simulink subsystem "GravityTorque"  (R2021a)
settings: Solver=VariableStepAuto  StartTime=0.0  StopTime=10.0  RelTol=1e-3
undefined symbols (not defined in the file): Isc, Ix, Iy, Iz, mu
libraries: aerolibutil x2, vrlib x1
settings Model: Creator=Laura  LastModifiedBy=Laura

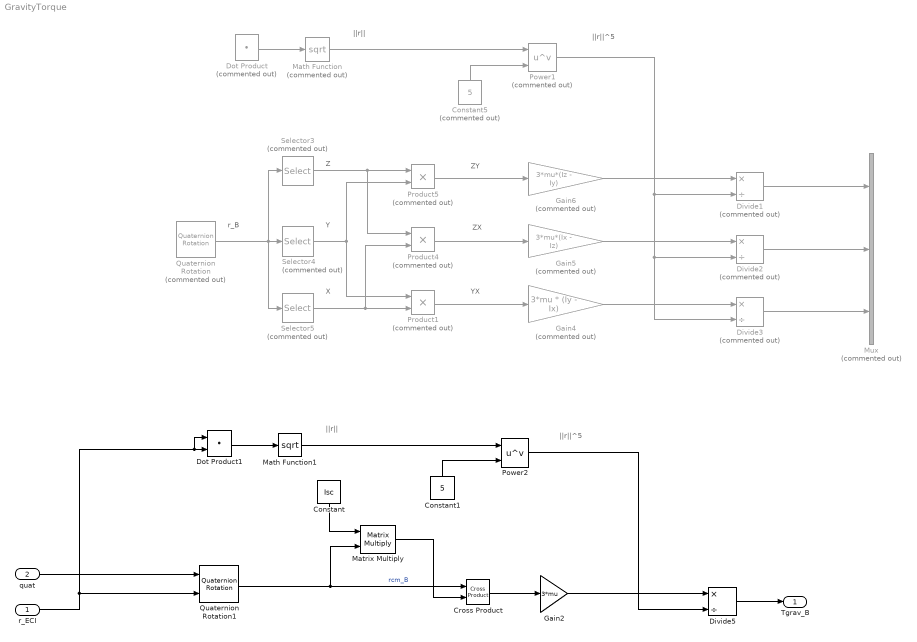
== system GravityTorque ==
  note: ||r||
  note: ||r||^5
  note: ||r||
  note: ZY
  note: Z
  note: ||r||^5
  note: YX
  note: Y
  note: ZX
  note: X
  note: r_B
  r_ECI : Inport
  quat : Inport  Port=2
  Constant : Constant  Value=Isc
  Constant1 : Constant  Value=5
  Constant5 : Constant  Commented=on  Value=5
  Cross Product : vrlib/Utilities/Cross Product
  Divide1 : Product  Commented=on  Inputs=*/
  Divide2 : Product  Commented=on  Inputs=*/
  Divide3 : Product  Commented=on  Inputs=*/
  Divide5 : Product  Inputs=*/
  Dot Product : DotProduct  Commented=on  InputSameDT=on  OutDataTypeStr=Inherit: Inherit via internal rule
  Dot Product1 : DotProduct  InputSameDT=on  OutDataTypeStr=Inherit: Inherit via internal rule
  Gain2 : Gain  Gain=3*mu
  Gain4 : Gain  Commented=on  Gain=3*mu * (Iy - Ix)
  Gain5 : Gain  Commented=on  Gain=3*mu*(Ix - Iz)
  Gain6 : Gain  Commented=on  Gain=3*mu*(Iz - Iy)
  Math Function : Math  Commented=on  Operator=sqrt  SignedPower=on  SaturateOnIntegerOverflow=on
  Math Function1 : Math  Operator=sqrt  SignedPower=on  SaturateOnIntegerOverflow=on
  Matrix Multiply : Product  Multiplication=Matrix(*)
  Mux : Mux  Commented=on  Inputs=3
  Power1 : Math  Commented=on  Operator=pow  SaturateOnIntegerOverflow=on
  Power2 : Math  Operator=pow  SaturateOnIntegerOverflow=on
  Product1 : Product  Commented=on
  Product4 : Product  Commented=on
  Product5 : Product  Commented=on
  Quaternion Rotation : aerolibutil/Quaternion Rotation  Commented=on
  Quaternion Rotation1 : aerolibutil/Quaternion Rotation
  Selector3 : Selector  Commented=on  InputPortWidth=3  IndexOptions=Index vector (dialog)  Indices=[3]  OutputSizes=1
  Selector4 : Selector  Commented=on  InputPortWidth=3  IndexOptions=Index vector (dialog)  Indices=[2]  OutputSizes=1
  Selector5 : Selector  Commented=on  InputPortWidth=3  IndexOptions=Index vector (dialog)  Indices=[1]  OutputSizes=1
  Tgrav_B : Outport  SampleTime=1
  wires:
  Cross Product/1 -> Gain2/1
  Matrix Multiply/1 -> Cross Product/2
  Constant/1 -> Matrix Multiply/1
  Quaternion Rotation1/1 -> Cross Product/1, Matrix Multiply/2  "rcm_B"
  r_ECI/1 -> Quaternion Rotation1/2, Dot Product1/1, Dot Product1/2
  Gain2/1 -> Divide5/1
  Math Function1/1 -> Power2/1
  Constant1/1 -> Power2/2
  Divide5/1 -> Tgrav_B/1
  Power2/1 -> Divide5/2
  Dot Product1/1 -> Math Function1/1
  quat/1 -> Quaternion Rotation1/1
  Divide3/1 -> Mux/3
  Divide2/1 -> Mux/2
  Divide1/1 -> Mux/1
  Power1/1 -> Divide1/2, Divide2/2, Divide3/2
  Math Function/1 -> Power1/1
  Dot Product/1 -> Math Function/1
  Product1/1 -> Gain4/1
  Product4/1 -> Gain5/1
  Gain5/1 -> Divide2/1
  Quaternion Rotation/1 -> Selector4/1, Selector3/1, Selector5/1
  Gain4/1 -> Divide3/1
  Selector5/1 -> Product4/2, Product1/2
  Selector3/1 -> Product4/1, Product5/1
  Selector4/1 -> Product5/2, Product1/1
  Constant5/1 -> Power1/2
  Product5/1 -> Gain6/1
  Gain6/1 -> Divide1/1
